simulink model "Ports"  (Simulink 7.7)
settings: Solver=ode45  StartTime=0.0  StopTime=10.0  RelTol=1e-3
libraries: orocos_taskcontext x30
settings Model: Creator=meyer  LastModifiedBy=meyer

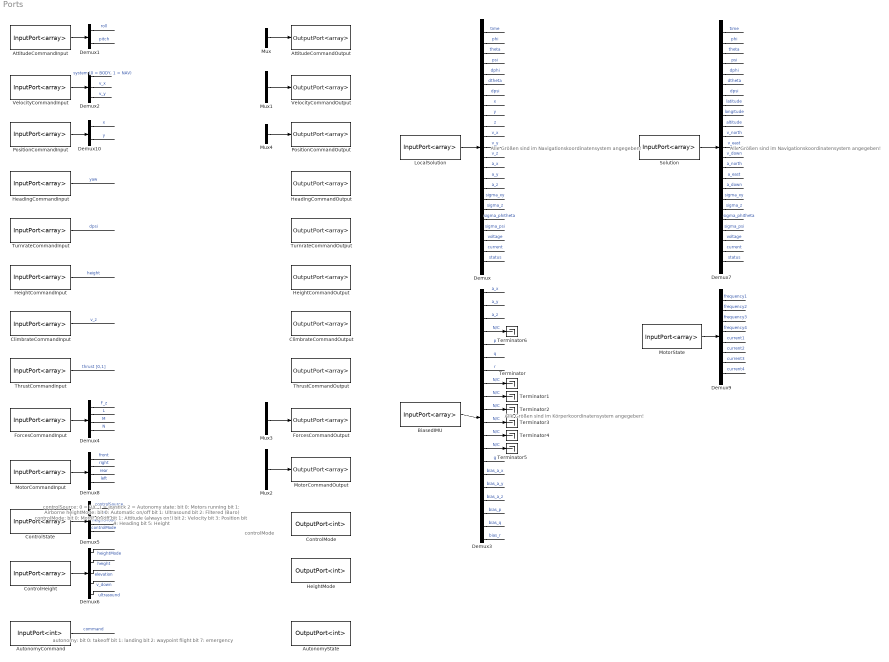
== system Ports ==
  note: Alle Größen sind im
      | Navigationskoordinatensystem angegeben!
  note: Alle Größen sind im
      | Körperkoordinatensystem angegeben!
  note: Alle Größen sind im
      | Navigationskoordinatensystem angegeben!
  note: controlSource:
      |   0 = R/C
      |   1 = Joystick
      |   2 = Autonomy
      | state:
      |   bit 0: Motors running
      |   bit 1: Airborne
      | heightMode:
      |   bit 0: Automatic on/off
      |   bit 1: Ultrasound
      |   bit 2: Filtered (Baro)
      | controlMode:
      |   bit 0: Motor on/off
      |   bit 1: Attitude (always on!)
      |   bit 2: Velocity
      |   bit 3: Position
      |   bit 4: Heading
      |   bit 5: Height
  note: autonomy:
      |   bit 0: takeoff
      |   bit 1: landing
      |   bit 2: waypoint flight
      |   bit 7: emergency
  note: controlMode
  AttitudeCommandInput : orocos_taskcontext/InputPort<array>  dpdesc=Port's Description  dpvalue=zeros(1,2)
      settings: AttributesFormatString=Value=%<dpvalue>
  AttitudeCommandOutput : orocos_taskcontext/OutputPort<array>  dpdesc=Port's Description  dpvalue=zeros(1,2)
      settings: AttributesFormatString=Value=%<dpvalue>
  AutonomyCommand : orocos_taskcontext/InputPort<int>  dpdesc=Port's Description  dpvalue=int32(0)
      settings: AttributesFormatString=Value=%<dpvalue>
  AutonomyState : orocos_taskcontext/OutputPort<int>  dpdesc=Port's Description  dpvalue=int32(0)
      settings: AttributesFormatString=Value=%<dpvalue>
  BiasedIMU : orocos_taskcontext/InputPort<array>  dpdesc=Port's Description  dpvalue=zeros(1,20)
      settings: AttributesFormatString=Value=%<dpvalue>
  ClimbrateCommandInput : orocos_taskcontext/InputPort<array>  dpdesc=Port's Description  dpvalue=0.0
      settings: AttributesFormatString=Value=%<dpvalue>
  ClimbrateCommandOutput : orocos_taskcontext/OutputPort<array>  dpdesc=Port's Description  dpvalue=0.0
      settings: AttributesFormatString=Value=%<dpvalue>
  ControlHeight : orocos_taskcontext/InputPort<array>  dpdesc=Port's Description  dpvalue=zeros(1,5)
      settings: AttributesFormatString=Value=%<dpvalue>
  ControlMode : orocos_taskcontext/OutputPort<int>  dpdesc=Port's Description  dpvalue=int32(0)
      settings: AttributesFormatString=Value=%<dpvalue>
  ControlState : orocos_taskcontext/InputPort<array>  dpdesc=Port's Description  dpvalue=zeros(1,4)
      settings: AttributesFormatString=Value=%<dpvalue>
  Demux : Demux  Outputs=23
  Demux1 : Demux  Outputs=2
  Demux10 : Demux  Outputs=2
  Demux2 : Demux  Outputs=3
  Demux3 : Demux  Outputs=20
  Demux4 : Demux
  Demux5 : Demux
  Demux6 : Demux  Outputs=5
  Demux7 : Demux  Outputs=23
  Demux8 : Demux
  Demux9 : Demux  Outputs=8
  ForcesCommandInput : orocos_taskcontext/InputPort<array>  dpdesc=Port's Description  dpvalue=zeros(1,4)
      settings: AttributesFormatString=Value=%<dpvalue>
  ForcesCommandOutput : orocos_taskcontext/OutputPort<array>  dpdesc=Port's Description  dpvalue=zeros(1,4)
      settings: AttributesFormatString=Value=%<dpvalue>
  HeadingCommandInput : orocos_taskcontext/InputPort<array>  dpdesc=Port's Description  dpvalue=0.0
      settings: AttributesFormatString=Value=%<dpvalue>
  HeadingCommandOutput : orocos_taskcontext/OutputPort<array>  dpdesc=Port's Description  dpvalue=0.0
      settings: AttributesFormatString=Value=%<dpvalue>
  HeightCommandInput : orocos_taskcontext/InputPort<array>  dpdesc=Port's Description  dpvalue=0.0
      settings: AttributesFormatString=Value=%<dpvalue>
  HeightCommandOutput : orocos_taskcontext/OutputPort<array>  dpdesc=Port's Description  dpvalue=0.0
      settings: AttributesFormatString=Value=%<dpvalue>
  HeightMode : orocos_taskcontext/OutputPort<int>  dpdesc=Port's Description  dpvalue=int32(0)
      settings: AttributesFormatString=Value=%<dpvalue>
  LocalSolution : orocos_taskcontext/InputPort<array>  dpdesc=Port's Description  dpvalue=zeros(1,23)
      settings: AttributesFormatString=Value=%<dpvalue>
  MotorCommandInput : orocos_taskcontext/InputPort<array>  dpdesc=Port's Description  dpvalue=zeros(1,4)
      settings: AttributesFormatString=Value=%<dpvalue>
  MotorCommandOutput : orocos_taskcontext/OutputPort<array>  dpdesc=Port's Description  dpvalue=zeros(1,4)
      settings: AttributesFormatString=Value=%<dpvalue>
  MotorState : orocos_taskcontext/InputPort<array>  dpdesc=Port's Description  dpvalue=zeros(1,8)
      settings: AttributesFormatString=Value=%<dpvalue>
  Mux : Mux  Inputs=2
  Mux1 : Mux  Inputs=3
  Mux2 : Mux
  Mux3 : Mux
  Mux4 : Mux  Inputs=2
  PositionCommandInput : orocos_taskcontext/InputPort<array>  dpdesc=Port's Description  dpvalue=zeros(1,2)
      settings: AttributesFormatString=Value=%<dpvalue>
  PositionCommandOutput : orocos_taskcontext/OutputPort<array>  dpdesc=Port's Description  dpvalue=zeros(1,2)
      settings: AttributesFormatString=Value=%<dpvalue>
  Solution : orocos_taskcontext/InputPort<array>  dpdesc=Port's Description  dpvalue=zeros(1,23)
      settings: AttributesFormatString=Value=%<dpvalue>
  Terminator{,1..6} (7 alike) : Terminator
  ThrustCommandInput : orocos_taskcontext/InputPort<array>  dpdesc=Port's Description  dpvalue=0.0
      settings: AttributesFormatString=Value=%<dpvalue>
  ThrustCommandOutput : orocos_taskcontext/OutputPort<array>  dpdesc=Port's Description  dpvalue=0.0
      settings: AttributesFormatString=Value=%<dpvalue>
  TurnrateCommandInput : orocos_taskcontext/InputPort<array>  dpdesc=Port's Description  dpvalue=0.0
      settings: AttributesFormatString=Value=%<dpvalue>
  TurnrateCommandOutput : orocos_taskcontext/OutputPort<array>  dpdesc=Port's Description  dpvalue=0.0
      settings: AttributesFormatString=Value=%<dpvalue>
  VelocityCommandInput : orocos_taskcontext/InputPort<array>  dpdesc=Port's Description  dpvalue=zeros(1,3)
      settings: AttributesFormatString=Value=%<dpvalue>
  VelocityCommandOutput : orocos_taskcontext/OutputPort<array>  dpdesc=Port's Description  dpvalue=zeros(1,3)
      settings: AttributesFormatString=Value=%<dpvalue>
  wires:
  Demux1/1 -> ?  "roll"
  Demux1/2 -> ?  "pitch"
  Demux/2 -> ?  "phi"
  Demux/1 -> ?  "time"
  Demux/3 -> ?  "theta"
  Demux/4 -> ?  "psi"
  Demux/5 -> ?  "dphi"
  Demux/6 -> ?  "dtheta"
  Demux/7 -> ?  "dpsi"
  Demux/8 -> ?  "x"
  Demux/9 -> ?  "y"
  Demux/10 -> ?  "z"
  Demux/11 -> ?  "v_x"
  Demux/12 -> ?  "v_y"
  Demux/13 -> ?  "v_z"
  HeadingCommandInput/1 -> ?  "yaw"
  Demux/14 -> ?  "a_x"
  Demux/15 -> ?  "a_y"
  Demux/16 -> ?  "a_z"
  Demux/17 -> ?  "sigma_xy"
  Demux/18 -> ?  "sigma_z"
  Demux/19 -> ?  "sigma_phitheta"
  Demux/20 -> ?  "sigma_psi"
  Demux/21 -> ?  "voltage"
  Demux/22 -> ?  "current"
  Demux/23 -> ?  "status"
  Mux/1 -> AttitudeCommandOutput/1
  ? -> Mux/1  "roll"
  ? -> Mux/2  "pitch"
  LocalSolution/1 -> Demux/1
  AttitudeCommandInput/1 -> Demux1/1
  ? -> HeadingCommandOutput/1  "yaw"
  HeightCommandInput/1 -> ?  "height"
  ClimbrateCommandInput/1 -> ?  "v_z"
  Demux2/2 -> ?  "v_x"
  Mux1/1 -> VelocityCommandOutput/1
  ? -> Mux1/1  "system"
  ? -> Mux1/2  "v_x"
  BiasedIMU/1 -> Demux3/1
  Demux3/1 -> ?  "a_x"
  Demux3/2 -> ?  "a_y"
  Demux3/3 -> ?  "a_z"
  Demux3/4 -> Terminator6/1  "N/C"
  Demux3/5 -> ?  "p"
  Demux3/6 -> ?  "q"
  Demux3/7 -> ?  "r"
  Demux3/8 -> Terminator/1  "N/C"
  Demux3/9 -> Terminator1/1  "N/C"
  Demux3/10 -> Terminator2/1  "N/C"
  Demux3/11 -> Terminator3/1  "N/C"
  Demux3/12 -> Terminator4/1  "N/C"
  Demux3/13 -> Terminator5/1  "N/C"
  Demux3/14 -> ?  "g"
  Demux3/15 -> ?  "bias_a_x"
  Demux3/16 -> ?  "bias_a_y"
  Demux3/17 -> ?  "bias_a_z"
  Demux3/18 -> ?  "bias_p"
  Demux3/19 -> ?  "bias_q"
  Demux3/20 -> ?  "bias_r"
  VelocityCommandInput/1 -> Demux2/1
  Demux2/3 -> ?  "v_y"
  Demux2/1 -> ?  "system (0 = BODY, 1 = NAV)"
  ? -> Mux1/3  "v_y"
  ThrustCommandInput/1 -> ?  "thrust [0,1]"
  ? -> HeightCommandOutput/1  "height"
  ? -> ClimbrateCommandOutput/1  "v_z"
  ? -> ThrustCommandOutput/1  "thrust [0,1]"
  Mux2/1 -> MotorCommandOutput/1
  ? -> Mux2/1  "front"
  ? -> Mux2/2  "right"
  ? -> Mux2/3  "rear"
  ? -> Mux2/4  "left"
  Mux3/1 -> ForcesCommandOutput/1
  ForcesCommandInput/1 -> Demux4/1
  Demux4/1 -> ?  "F_z"
  Demux4/2 -> ?  "L"
  Demux4/3 -> ?  "M"
  Demux4/4 -> ?  "N"
  ? -> Mux3/1  "F_z"
  ? -> Mux3/2  "L"
  ? -> Mux3/3  "M"
  ? -> Mux3/4  "N"
  Demux5/1 -> ?  "controlSource"
  Demux5/3 -> ?  "heightMode"
  Demux5/4 -> ?  "controlMode"
  ControlState/1 -> Demux5/1
  Demux6/1 -> ?  "heightMode"
  Demux6/2 -> ?  "height"
  Demux6/3 -> ?  "elevation"
  Demux6/4 -> ?  "v_down"
  ControlHeight/1 -> Demux6/1
  TurnrateCommandInput/1 -> ?  "dpsi"
  ? -> TurnrateCommandOutput/1  "dpsi"
  Demux7/2 -> ?  "phi"
  Demux7/1 -> ?  "time"
  Demux7/3 -> ?  "theta"
  Demux7/4 -> ?  "psi"
  Demux7/5 -> ?  "dphi"
  Demux7/6 -> ?  "dtheta"
  Demux7/7 -> ?  "dpsi"
  Demux7/8 -> ?  "latitude"
  Demux7/9 -> ?  "longitude"
  Demux7/10 -> ?  "altitude"
  Demux7/11 -> ?  "v_north"
  Demux7/12 -> ?  "v_east"
  Demux7/13 -> ?  "v_down"
  Demux7/14 -> ?  "a_north"
  Demux7/15 -> ?  "a_east"
  Demux7/16 -> ?  "a_down"
  Demux7/17 -> ?  "sigma_xy"
  Demux7/18 -> ?  "sigma_z"
  Demux7/19 -> ?  "sigma_phitheta"
  Demux7/20 -> ?  "sigma_psi"
  Demux7/21 -> ?  "voltage"
  Demux7/22 -> ?  "current"
  Demux7/23 -> ?  "status"
  Solution/1 -> Demux7/1
  MotorCommandInput/1 -> Demux8/1
  Demux8/1 -> ?  "front"
  Demux8/2 -> ?  "right"
  Demux8/3 -> ?  "rear"
  Demux8/4 -> ?  "left"
  MotorState/1 -> Demux9/1
  Demux9/1 -> ?  "frequency1"
  Demux9/2 -> ?  "frequency2"
  Demux9/3 -> ?  "frequency3"
  Demux9/4 -> ?  "frequency4"
  Demux9/5 -> ?  "current1"
  Demux9/6 -> ?  "current2"
  Demux9/7 -> ?  "current3"
  Demux9/8 -> ?  "current4"
  PositionCommandInput/1 -> Demux10/1
  Demux10/1 -> ?  "x"
  Demux10/2 -> ?  "y"
  Mux4/1 -> PositionCommandOutput/1
  ? -> Mux4/1  "x"
  ? -> Mux4/2  "y"
  AutonomyCommand/1 -> ?  "command"
  ? -> AutonomyState/1  "state"
  Demux5/2 -> ?  "state"
  Demux6/5 -> ?  "ultrasound"
  ? -> HeightMode/1  "heightMode"
  ? -> ControlMode/1
